simulink model "test_pid"  (R2024a)
settings: Solver=VariableStepAuto  StartTime=0.0  StopTime=120  RelTol=1e-3
settings Model: Creator=sabri  LastModifiedBy=sabri

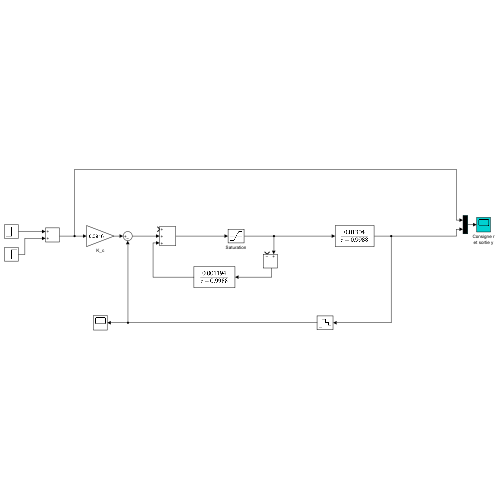
[thumbnail: Simulink's stored preview of the top-level diagram]
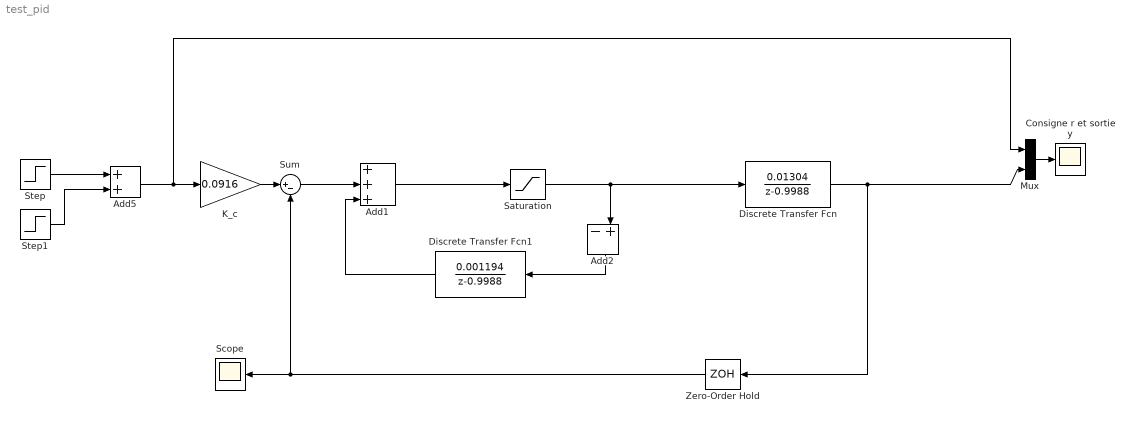
== system test_pid ==
  Add1 : Sum  Inputs=+++
  Add2 : Sum  Inputs=-+
  Add5 : Sum
  Consigne r et sortie y : Scope
  Discrete Transfer Fcn : DiscreteTransferFcn  Numerator=[0.01304]  Denominator=[1 -0.9988]
  Discrete Transfer Fcn1 : DiscreteTransferFcn  Numerator=[0.001194]  Denominator=[1 -0.9988]
  K_c : Gain  Gain=0.0916
  Mux : Mux  Inputs=2
  Saturation : Saturate  UpperLimit=50  LowerLimit=0
  Scope : Scope
  Step : Step  Time=10  After=10  SampleTime=0
  Step1 : Step  Time=60  After=0  SampleTime=0
  Sum : Sum  Inputs=|+-
  Zero-Order Hold : ZeroOrderHold  SampleTime=0.1
  wires:
  Add5/1 -> Mux/1, K_c/1
  Discrete Transfer Fcn/1 -> Mux/2, Zero-Order Hold/1
  Mux/1 -> Consigne r et sortie y/1
  Step/1 -> Add5/1
  Step1/1 -> Add5/2
  Saturation/1 -> Discrete Transfer Fcn/1, Add2/2
  Sum/1 -> Add1/2
  Add1/1 -> Saturation/1
  Discrete Transfer Fcn1/1 -> Add1/3
  Add2/1 -> Discrete Transfer Fcn1/1
  K_c/1 -> Sum/1
  Zero-Order Hold/1 -> Sum/2, Scope/1
